simulink model "CA2"  (R2023b)
settings: Solver=VariableStepAuto  StartTime=0.0  StopTime=20  RelTol=1e-3
settings Model: Creator=shipingguo  LastModifiedBy=shipingguo

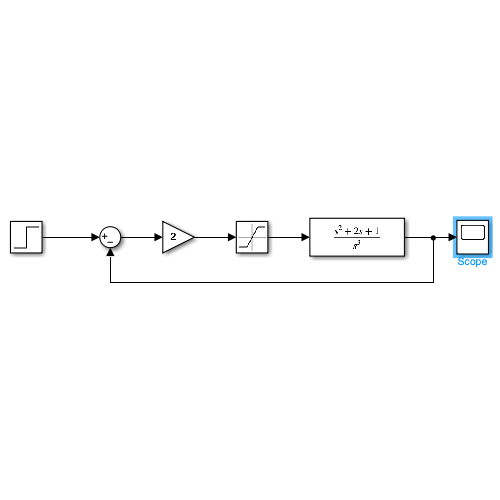
[thumbnail: Simulink's stored preview of the top-level diagram]
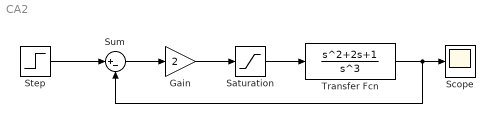
== system CA2 ==
  Gain : Gain  Gain=2
  Saturation : Saturate  UpperLimit=1  LowerLimit=-1
  Scope : Scope
  Step : Step  After=4  SampleTime=0
  Sum : Sum  Inputs=|+-
  Transfer Fcn : TransferFcn  Numerator=[1, 2, 1]  Denominator=[1, 0, 0, 0]
  wires:
  Saturation/1 -> Transfer Fcn/1
  Step/1 -> Sum/1
  Sum/1 -> Gain/1
  Gain/1 -> Saturation/1
  Transfer Fcn/1 -> Scope/1, Sum/2
